simulink library "ESTS_UOD_CornrgDir"  (R2022a)
settings: Solver=VariableStepAuto  StartTime=0.0  StopTime=10.0  RelTol=1e-3
undefined symbols (not defined in the file or in its folder): ESTS_UOD_c_TiSample_s, ESTS_UOD_p_SwtTimDel_s, ESTS_UOD_p_TimDel_s
libraries: VUT_lib x4
settings Model: Creator=blatak  LastModifiedBy=blatak

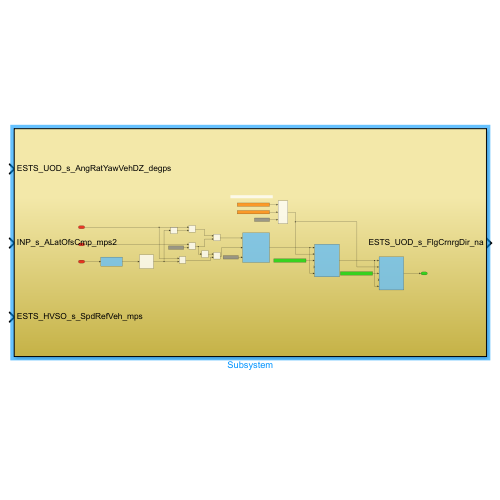
[thumbnail: Simulink's stored preview of the top-level diagram]
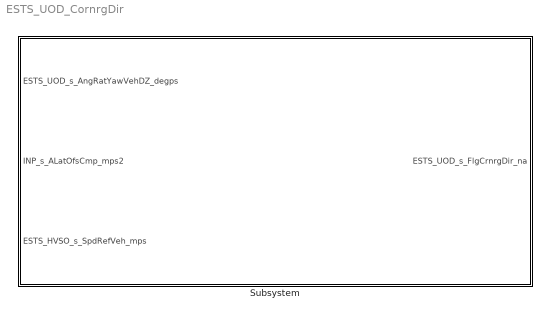
== system ESTS_UOD_CornrgDir ==
  Subsystem : Subsystem

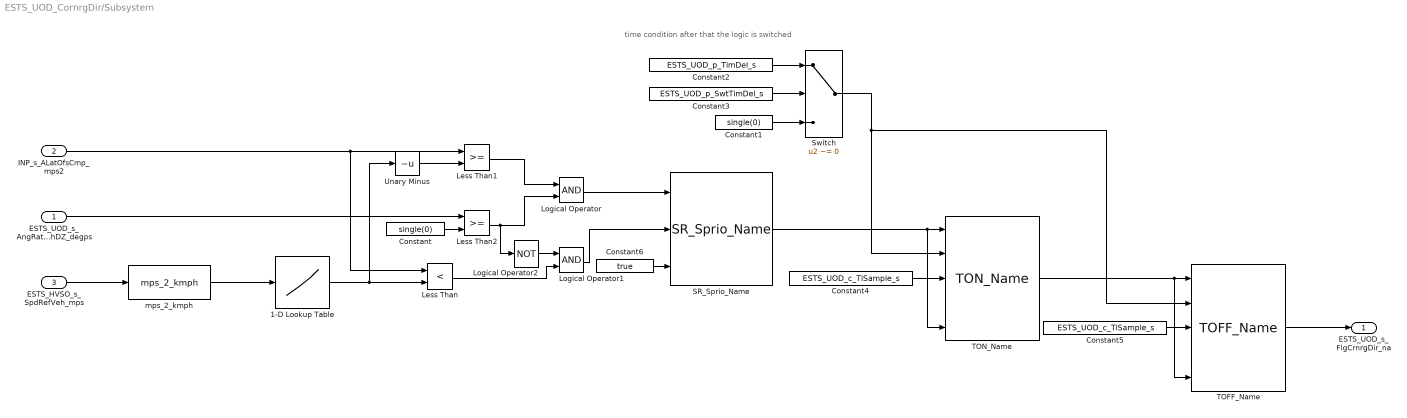
== system ESTS_UOD_CornrgDir/Subsystem ==
  note: time condition after that the logic is switched
  ESTS_UOD_s_AngRatYawVehDZ_degps : Inport
  INP_s_ALatOfsCmp_mps2 : Inport  Port=2
  ESTS_HVSO_s_SpdRefVeh_mps : Inport  Port=3
  1-D Lookup Table : Lookup_n-D  NumberOfTableDimensions=1  BreakpointsForDimension1=[-5:5]  Table=tanh([-5:5])  InternalRulePriority=Speed  RndMeth=Simplest
  Constant : Constant  Value=single(0)
  Constant1 : Constant  Value=single(0)
  Constant2 : Constant  Value=ESTS_UOD_p_TimDel_s
  Constant3 : Constant  Value=ESTS_UOD_p_SwtTimDel_s
  Constant4 : Constant  Value=ESTS_UOD_c_TiSample_s
  Constant5 : Constant  Value=ESTS_UOD_c_TiSample_s
  Constant6 : Constant  Value=true  OutDataTypeStr=boolean
  Less Than : RelationalOperator  Operator=<  OutDataTypeStr=boolean  RndMeth=Simplest  InputSameDT=off
  Less Than1 : RelationalOperator  OutDataTypeStr=boolean  RndMeth=Simplest  InputSameDT=off
  Less Than2 : RelationalOperator  OutDataTypeStr=boolean  RndMeth=Simplest  InputSameDT=off
  Logical Operator : Logic  AllPortsSameDT=off  OutDataTypeStr=boolean
  Logical Operator1 : Logic  AllPortsSameDT=off  OutDataTypeStr=boolean
  Logical Operator2 : Logic  Operator=NOT  AllPortsSameDT=off  OutDataTypeStr=boolean
  SR_Sprio_Name : VUT_lib/SR_Sprio_Name  SystemSampleTime=-1  VariantActivationTime=update diagram  Latency=0  AutoFrameSizeCalculation=off
  Switch : Switch  Criteria=u2 ~= 0  SaturateOnIntegerOverflow=off  InputSameDT=off
  TOFF_Name : VUT_lib/TOFF_Name  SystemSampleTime=-1  VariantActivationTime=update diagram  Latency=0  AutoFrameSizeCalculation=off
  TON_Name : VUT_lib/TON_Name  SystemSampleTime=-1  VariantActivationTime=update diagram  Latency=0  AutoFrameSizeCalculation=off
  Unary Minus : UnaryMinus
  mps_2_kmph : VUT_lib/mps_2_kmph  SystemSampleTime=-1  VariantActivationTime=update diagram  Latency=0  AutoFrameSizeCalculation=off
  ESTS_UOD_s_FlgCrnrgDir_na : Outport
  wires:
  1-D Lookup Table/1 -> Unary Minus/1, Less Than/2
  ESTS_UOD_s_AngRatYawVehDZ_degps/1 -> Less Than2/1
  Less Than2/1 -> Logical Operator2/1, Logical Operator/2
  Logical Operator1/1 -> SR_Sprio_Name/2
  Constant6/1 -> SR_Sprio_Name/3
  mps_2_kmph/1 -> 1-D Lookup Table/1
  TON_Name/1 -> TOFF_Name/5, TOFF_Name/1
  Constant/1 -> Less Than2/2
  Constant5/1 -> TOFF_Name/3
  Less Than1/1 -> Logical Operator/1
  SR_Sprio_Name/1 -> TON_Name/5, TON_Name/1
  Switch/1 -> TON_Name/2, TOFF_Name/2
  ESTS_HVSO_s_SpdRefVeh_mps/1 -> mps_2_kmph/1
  Constant1/1 -> Switch/3
  Less Than/1 -> Logical Operator1/2
  Logical Operator2/1 -> Logical Operator1/1
  TOFF_Name/1 -> ESTS_UOD_s_FlgCrnrgDir_na/1
  INP_s_ALatOfsCmp_mps2/1 -> Less Than/1, Less Than1/1
  Constant2/1 -> Switch/1
  Logical Operator/1 -> SR_Sprio_Name/1
  Unary Minus/1 -> Less Than1/2
  Constant4/1 -> TON_Name/3
  Constant3/1 -> Switch/2
